simulink model "smart_door_sim"  (R2021a)
settings: Solver=VariableStepAuto  StartTime=0.0  StopTime=10  RelTol=1e-3
values from neighbouring files (symbols this model uses):
  entered_pin = zeros(1,4)    [smart_door_3d_simulation_pro.m]
libraries: simulink x4
settings Model: Creator=samad  LastModifiedBy=samad

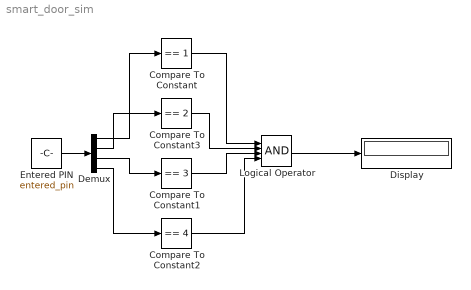
== system smart_door_sim ==
  Compare To Constant : simulink/Logic and Bit Operations/Compare To Constant  relop===  const=1  OutDataTypeStr=boolean
  Compare To Constant1 : simulink/Logic and Bit Operations/Compare To Constant  relop===  const=3  OutDataTypeStr=boolean
  Compare To Constant2 : simulink/Logic and Bit Operations/Compare To Constant  relop===  const=4  OutDataTypeStr=boolean
  Compare To Constant3 : simulink/Logic and Bit Operations/Compare To Constant  relop===  const=2  OutDataTypeStr=boolean
  Demux : Demux
  Display : Display
  Entered PIN : Constant  Value=entered_pin  OutDataTypeStr=double
  Logical Operator : Logic  Inputs=4  AllPortsSameDT=off  OutDataTypeStr=boolean
  wires:
  Demux/1 -> Compare To Constant/1
  Demux/3 -> Compare To Constant1/1
  Demux/2 -> Compare To Constant3/1
  Demux/4 -> Compare To Constant2/1
  Entered PIN/1 -> Demux/1
  Compare To Constant/1 -> Logical Operator/1
  Compare To Constant3/1 -> Logical Operator/2
  Compare To Constant1/1 -> Logical Operator/3
  Compare To Constant2/1 -> Logical Operator/4
  Logical Operator/1 -> Display/1
